simulink library "LibraryFM"  (R2016b)
settings: Solver=VariableStepAuto  StartTime=0.0  StopTime=10.0  RelTol=1e-3
undefined symbols (not defined in the file or in its folder): ActuatorStruct, drivePeakCurrent, FM1, Lb, Lf, Lu, motorTorqueConstant, RobotStruct, sampleTime, transmissionRatio
undefined symbols (not defined in the file): JointAbsoluteEncoderCounts_rev
libraries: simulink x34, LibraryFM x13, VariousBlocksLibrary x4, dspstat3 x1, simulink_extras x1, FM_Library x1
(part 2 of 3)

== system LibraryFM/DataToEtherCAT/WorkspacePositionGuard ==
  note: Check for singularity of joint configuration by checking
      | the condition number. When it exceeds a certain value, go to a safe mode
      | For now, this means disabling the actuators.
      | Note that the boundaries set using admittance should prohibit this from happening.
      | However, if sometjhing really goes wrong, this is a safe guard
  note: Check whether endpoint position is within the predefined workspace
      | (ellipse)
  note: Check internal angles
  BusRobot : Inport
  StateSystem : Inport  Port=2
  AvoidAlgebraicLoop : Memory
  Bus Selector : BusSelector  OutputSignals=xOpSpace.x,xOpSpace.jacobian,qJointSpace.q_all
  CheckForSingularity : MATLAB Function  TreatAsAtomicUnit=on
  CheckInternalAngles : MATLAB Function  TreatAsAtomicUnit=on
  Compare To Constant : simulink/Logic and Bit Operations/Compare To Constant  relop===  const=4  OutDataTypeStr=boolean
  Compare To Constant1 : simulink/Logic and Bit Operations/Compare To Constant  relop=>=  const=120  OutDataTypeStr=boolean
  CreateSingleErrorValue : LibraryFM/ToActuator1/DriveEnableLogic/CreateSingleErrorValue
  Data Type Conversion1 : DataTypeConversion  OutDataTypeStr=boolean
  Data Type Conversion2 : DataTypeConversion  Commented=through  OutDataTypeStr=int32
  Data Type Conversion4 : DataTypeConversion  OutDataTypeStr=boolean
  Detect Change : simulink/Logic and Bit Operations/Detect Change  vinit=0  InputProcessing=Inherited  OutDataTypeStr=boolean
  EndpointPositionGuard : MATLAB Function  TreatAsAtomicUnit=on
  LatchRising : LibraryFM/Utilities/LatchRising  ic=0
  Mux : Mux  Inputs=3
  ShowWorkspaceErrorLatched : Display
  WorkspaceLastError : Display
  WorkspaceError : Outport
  WorkspaceErrorLatched : Outport  Port=2
  wires:
  Data Type Conversion4/1 -> Mux/3
  Bus Selector/3 -> CheckInternalAngles/1(theta)  "<q_all>"
  CheckInternalAngles/1(angleError) -> Data Type Conversion4/1
  Compare To Constant1/1 -> Mux/2
  Data Type Conversion1/1 -> Mux/1
  Data Type Conversion2/1 -> WorkspaceErrorLatched/1, ShowWorkspaceErrorLatched/1
  StateSystem/1 -> Compare To Constant/1
  Bus Selector/2 -> CheckForSingularity/1(J)  "<jacobian>"
  Compare To Constant/1 -> EndpointPositionGuard/2(correctState)
  AvoidAlgebraicLoop/1 -> WorkspaceError/1, Detect Change/1, LatchRising/1
  Detect Change/1 -> LatchRising/Trigger
  CreateSingleErrorValue/1 -> AvoidAlgebraicLoop/1
  EndpointPositionGuard/1(error) -> Data Type Conversion1/1
  LatchRising/1 -> Data Type Conversion2/1
  Bus Selector/1 -> EndpointPositionGuard/1(xe)  "<x>"
  BusRobot/1 -> Bus Selector/1
  Mux/1 -> WorkspaceLastError/1, CreateSingleErrorValue/1
  CheckForSingularity/1(kappa) -> Compare To Constant1/1

== system LibraryFM/DriveEnableLogic1/16_TorqueGuard ==
  BusActuator : Inport
  TorqueGuardMax : Inport  Port=2
  Abs : Abs
  Bus Selector : BusSelector  OutputSignals=JointTorque_Act_Nm
  Relational Operator : RelationalOperator  Operator=>  OutDataTypeStr=boolean  RndMeth=Nearest
  Error : Outport
  wires:
  Relational Operator/1 -> Error/1
  Abs/1 -> Relational Operator/1
  BusActuator/1 -> Bus Selector/1
  Bus Selector/1 -> Abs/1  "<JointTorque_Act_Nm>"
  TorqueGuardMax/1 -> Relational Operator/2

== system LibraryFM/DriveEnableLogic1/1_ActuatorNotInUse ==
  note: When UseActuator = 0, this block outputs 1. Later in the chain, the ErrorValue is then negated, resulting in -1 if there are no other errors. Note, thus, that this output does not really indicate an error; more a status.
  UseActuator : Inport
  Logical Operator1 : Logic  Operator=NOT  AllPortsSameDT=off  OutDataTypeStr=boolean
  Error : Outport
  wires:
  UseActuator/1 -> Logical Operator1/1
  Logical Operator1/1 -> Error/1

== system LibraryFM/DriveEnableLogic1/2_JointAnglePositionGuard ==
  note: This block makes sure that the motors are turned off (and cannot go on) when the joint is outside its normal range.
  BusActuator : Inport
  Bus Selector : BusSelector  OutputSignals=JointPosition_rad
  Logical Operator : Logic  Operator=OR  AllPortsSameDT=off  OutDataTypeStr=boolean
  Maximum : Constant  Value=ActuatorStruct.JointPositionGuardMax
  Minimum : Constant  Value=ActuatorStruct.JointPositionGuardMin
  Relational Operator : RelationalOperator  Operator=<=  OutDataTypeStr=boolean  RndMeth=Nearest
  Relational Operator1 : RelationalOperator  OutDataTypeStr=boolean  RndMeth=Nearest
  Error : Outport
  wires:
  Bus Selector/1 -> Relational Operator/1, Relational Operator1/1  "<JointPosition_rad>"
  Maximum/1 -> Relational Operator1/2
  Minimum/1 -> Relational Operator/2
  Logical Operator/1 -> Error/1
  Relational Operator1/1 -> Logical Operator/2
  Relational Operator/1 -> Logical Operator/1
  BusActuator/1 -> Bus Selector/1

== system LibraryFM/DriveEnableLogic1/32_DriveError ==
  note: This block checks whether the drive went off by itself. Reasons why this could happen are: undervoltage of the motor power supply, short-circuit detection triggered, I2t error etc.
      | The first few seconds that the drive should be on (i.e., DriveEnable = True), the drive is in the process of turning on, and will not be really on. In order to avoid direct turn-off due to this, we disable this error the first few seconds.
  note: This memory block is to avoid an
      | algebraic loop
  note: This memory block is to avoid that this error 'turns on' when another error is triggered.
  BusActuator : Inport
  DriveEnable : Inport  Port=2
  Bus Selector : BusSelector  OutputSignals=OperationEnabled
  CountHowLongEnableWasTrue : MATLAB Function  TreatAsAtomicUnit=on
  InhibitTime_s : Constant  Value=2.0
  Logical Operator : Logic  AllPortsSameDT=off  OutDataTypeStr=boolean
  Logical Operator2 : Logic  Operator=NOT  AllPortsSameDT=off  OutDataTypeStr=boolean
  Memory : Memory
  Memory1 : Memory
  Relational Operator : RelationalOperator  OutDataTypeStr=boolean  RndMeth=Nearest
  ToSeconds : Gain  Gain=sampleTime
  Error : Outport
  wires:
  Logical Operator2/1 -> Logical Operator/2
  Memory1/1 -> Bus Selector/1
  Memory/1 -> CountHowLongEnableWasTrue/1(u)
  InhibitTime_s/1 -> Relational Operator/2
  Relational Operator/1 -> Logical Operator/1
  ToSeconds/1 -> Relational Operator/1
  CountHowLongEnableWasTrue/1(y) -> ToSeconds/1
  DriveEnable/1 -> Memory/1
  Bus Selector/1 -> Logical Operator2/1  "<OperationEnabled>"
  BusActuator/1 -> Memory1/1
  Logical Operator/1 -> Error/1

== system LibraryFM/DriveEnableLogic1/4_TransmissionSlip ==
  note: This block makes sure that the motors are turned off when the transmission slips.
  BusActuator : Inport
  Abs : Abs
  Bus Selector : BusSelector  OutputSignals=JointPosition_rad,JointPosition_AbsEnc_rad
  Minimum : Constant  Value=ActuatorStruct.TransmissionSlipAngleGuardMax
  Relational Operator1 : RelationalOperator  OutDataTypeStr=boolean  RndMeth=Nearest
  Slip : Display
  Subtract : Sum  Inputs=+-
  Error : Outport
  wires:
  Abs/1 -> Relational Operator1/1
  Bus Selector/1 -> Subtract/1  "<JointPosition_rad>"
  BusActuator/1 -> Bus Selector/1
  Minimum/1 -> Relational Operator1/2
  Bus Selector/2 -> Subtract/2  "<JointPosition_AbsEnc_rad>"
  Subtract/1 -> Abs/1, Slip/1
  Relational Operator1/1 -> Error/1

== system LibraryFM/DriveEnableLogic1/8_JointVelocityGuard ==
  To_ToActuator : Inport
  Abs : Abs
  Bus Selector : BusSelector  OutputSignals=JointPosition_rad
  Constant : Constant  Value=2*pi
  LPF Diff : Subsystem
  Relational Operator : RelationalOperator  OutDataTypeStr=boolean  RndMeth=Simplest
  Error : Outport
  wires:
  To_ToActuator/1 -> Bus Selector/1
  Bus Selector/1 -> LPF Diff/1(JointPosition_rad)  "<JointPosition_rad>"
  LPF Diff/1(JointVelocity_LPF_rads) -> Abs/1
  Abs/1 -> Relational Operator/1
  Constant/1 -> Relational Operator/2
  Relational Operator/1 -> Error/1

== system LibraryFM/DriveEnableLogic1/LatchRising ==
  in : Inport
  Trigger : TriggerPort  VariantControl=Variant  PortDimensions=1
  out : Outport
  wires:
  in/1 -> out/1

== system LibraryFM/FromActuator1/CalculateJointVelocity ==
  JointPosition_rad : Inport
  FOAW : MATLAB Function  Commented=on  TreatAsAtomicUnit=on
  Gain : Gain  Commented=on
  LPF Diff - 2nd order : LibraryFM/LPF Diff - 2nd order
  encoder noise : Constant  Commented=on  Value=ActuatorStruct.FOAWNoiseLevel
  JointVelocity_rads : Outport
  JointVelocity_LPF_rads : Outport  Port=2
  wires:
  JointPosition_rad/1 -> LPF Diff - 2nd order/1
  LPF Diff - 2nd order/1 -> JointVelocity_rads/1, JointVelocity_LPF_rads/1
  encoder noise/1 -> Gain/1
  Gain/1 -> FOAW/2(noise)

== system LibraryFM/PD + AFFC/AFFC ==
  q_ref : Inport
  qdot_ref : Inport  Port=2
  qddot_ref : Inport  Port=3
  e : Inport  Port=4
  Enable : EnablePort  StatesWhenEnabling=reset
  AFFC : MATLAB Function  TreatAsAtomicUnit=on
  Counter Free-Running : simulink/Sources/Counter Free-Running  NumBits=32  tsamp=-1
  Data Type Conversion : DataTypeConversion  OutDataTypeStr=double
  Learning factors : Constant  Value=[1e-5;5e-3;5e-4;1e-3]
  sample time : Gain  Gain=sampleTime
  p : Outport  OutputWhenDisabled=reset  InitialOutput=zeros(7,1)
  tau_affc : Outport  Port=2  OutputWhenDisabled=reset  InitialOutput=[0;0]
  wires:
  Learning factors/1 -> AFFC/6(w)
  Data Type Conversion/1 -> sample time/1
  sample time/1 -> AFFC/1(t)
  Counter Free-Running/1 -> Data Type Conversion/1
  AFFC/1(p) -> p/1
  AFFC/2(tau) -> tau_affc/1
  q_ref/1 -> AFFC/2(q)
  qdot_ref/1 -> AFFC/3(qdot)
  qddot_ref/1 -> AFFC/4(qddot)
  e/1 -> AFFC/5(e)

== system LibraryFM/ToActuator1/AppendToBus ==
  Bus_in : Inport
  DriveError : Inport  Port=2
  DesiredTorque : Inport  Port=3
  DesiredTorqueLimited : Inport  Port=4
  Bus Creator : BusCreator  Inputs=12
  Bus Selector2 : BusSelector  OutputSignals=OperationEnabled,StatusWord,JointPosition_IncEnc_rad,JointVelocity_LPF_rads,MotorEncoder_counts,MotorPosition_IncEnc_rad,JointAbsoluteEncoder_counts,JointTorque_Act_Nm,JointPosition_AbsEnc_rad
  Data Type Conversion : DataTypeConversion  OutDataTypeStr=double
  Bus_out : Outport
  wires:
  Bus Selector2/8 -> Bus Creator/8  "<JointTorque_Act_Nm>"
  Bus Creator/1 -> Bus_out/1
  Bus_in/1 -> Bus Selector2/1
  DriveError/1 -> Data Type Conversion/1
  Data Type Conversion/1 -> Bus Creator/12  "DriveError"
  DesiredTorque/1 -> Bus Creator/10  "DesiredTorque_Nm"
  DesiredTorqueLimited/1 -> Bus Creator/11  "DesiredTorqueLimited_Nm"
  Bus Selector2/1 -> Bus Creator/1  "<OperationEnabled>"
  Bus Selector2/2 -> Bus Creator/2  "<StatusWord>"
  Bus Selector2/3 -> Bus Creator/3  "<JointPosition_IncEnc_rad>"
  Bus Selector2/4 -> Bus Creator/4  "<JointVelocity_LPF_rads>"
  Bus Selector2/5 -> Bus Creator/5  "<MotorEncoder_counts>"
  Bus Selector2/7 -> Bus Creator/7  "<JointAbsoluteEncoder_counts>"
  Bus Selector2/6 -> Bus Creator/6  "<MotorPosition_IncEnc_rad>"
  Bus Selector2/9 -> Bus Creator/9  "<JointPosition_AbsEnc_rad>"

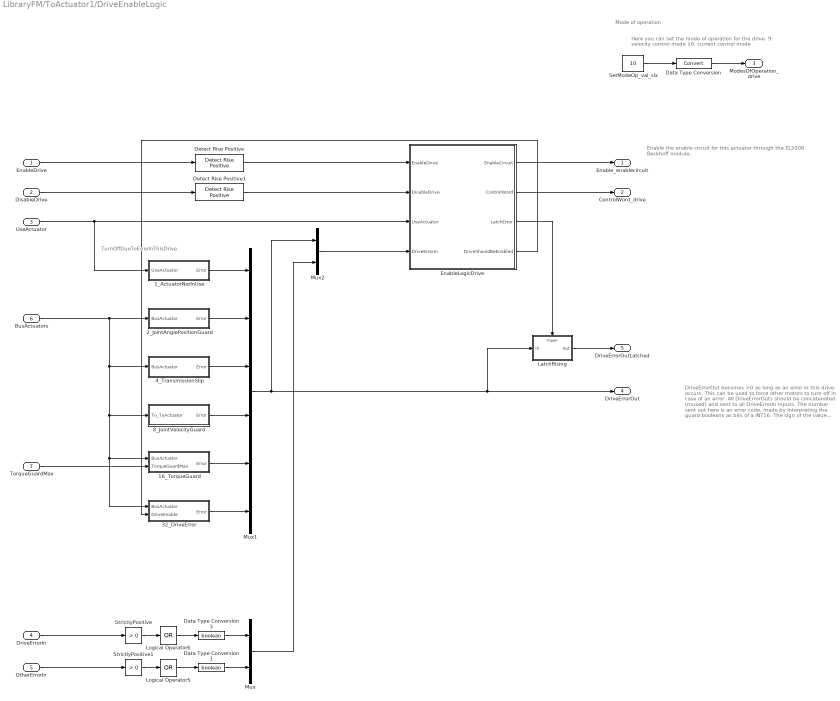
== system LibraryFM/ToActuator1/DriveEnableLogic ==
  note: Mode of operation
  note: Here you can set the mode of operation for the drive.
      | 9: velocity control mode
      | 10: current control mode
  note: TurnOffDueToErrorInThisDrive
  note: DriveErrorOut becomes >0 as long as an error in this drive occurs. This can be used to force other motors to turn off in case of an error.
      | All DriveErrorOuts should be concatenated (muxed)  and sent to all DriveErrorIn inputs. The number sent out here is an error code, made by interpreting the guard booleans as bits of a INT16.
      | The sign of the value indicates:
      | >=0: UseActuator=true
      | <0: UseActuator = False
  note: Enable the enable circuit for this actuator through the EL2008
      | Beckhoff module.
  EnableDrive : Inport
  DisableDrive : Inport  Port=2
  UseActuator : Inport  Port=3
  DriveErrorIn : Inport  Port=4
  OtherErrorIn : Inport  Port=5
  BusActuators : Inport  Port=6
  TorqueGuardMax : Inport  Port=7
  16_TorqueGuard : Subsystem
  1_ActuatorNotInUse : Subsystem
  2_JointAnglePositionGuard : Subsystem
  32_DriveError : Subsystem
  4_TransmissionSlip : Subsystem
  8_JointVelocityGuard : Subsystem
  Data Type Conversion : DataTypeConversion
  Data Type Conversion1 : DataTypeConversion  OutDataTypeStr=boolean
  Data Type Conversion3 : DataTypeConversion  OutDataTypeStr=boolean
  Detect Rise Positive : simulink/Logic and Bit Operations/Detect Rise Positive  vinit=0  InputProcessing=Inherited  OutDataTypeStr=boolean
  Detect Rise Positive1 : simulink/Logic and Bit Operations/Detect Rise Positive  vinit=0  InputProcessing=Inherited  OutDataTypeStr=boolean
  EnableLogicDrive : Subsystem
  LatchRising : Subsystem  TreatAsAtomicUnit=on
  Logical Operator5 : Logic  Operator=OR  Inputs=1  AllPortsSameDT=off  OutDataTypeStr=boolean
  Logical Operator6 : Logic  Operator=OR  Inputs=1  AllPortsSameDT=off  OutDataTypeStr=boolean
  Mux : Mux  Inputs=2
  Mux1 : Mux  Inputs=6
  Mux2 : Mux  Inputs=2
  SetModeOp_val_slx : Constant  Value=10
  StrictlyPositive : simulink/Logic and Bit Operations/Compare To Zero  relop=>  OutDataTypeStr=boolean
  StrictlyPositive1 : simulink/Logic and Bit Operations/Compare To Zero  relop=>  OutDataTypeStr=boolean
  Enable_enablecircuit : Outport
  ControlWord_drive : Outport  Port=2
  ModesOfOperation_drive : Outport  Port=3
  DriveErrorOut : Outport  Port=4
  DriveErrorOutLatched : Outport  Port=5
  wires:
  Mux/1 -> Mux2/2
  OtherErrorIn/1 -> StrictlyPositive1/1
  Logical Operator5/1 -> Data Type Conversion1/1
  Data Type Conversion3/1 -> Mux/1
  16_TorqueGuard/1(Error) -> Mux1/5
  32_DriveError/1(Error) -> Mux1/6
  1_ActuatorNotInUse/1(Error) -> Mux1/1
  BusActuators/1 -> 4_TransmissionSlip/1(BusActuator), 8_JointVelocityGuard/1(To_ToActuator), 32_DriveError/1(BusActuator), 16_TorqueGuard/1(BusActuator), 2_JointAnglePositionGuard/1(BusActuator)
  Logical Operator6/1 -> Data Type Conversion3/1
  DriveErrorIn/1 -> StrictlyPositive/1
  UseActuator/1 -> 1_ActuatorNotInUse/1(UseActuator), EnableLogicDrive/3(UseActuator)
  Data Type Conversion/1 -> ModesOfOperation_drive/1
  DisableDrive/1 -> Detect Rise Positive1/1
  Detect Rise Positive1/1 -> EnableLogicDrive/2(DisableDrive)
  EnableDrive/1 -> Detect Rise Positive/1
  SetModeOp_val_slx/1 -> Data Type Conversion/1
  TorqueGuardMax/1 -> 16_TorqueGuard/2(TorqueGuardMax)
  StrictlyPositive/1 -> Logical Operator6/1
  Mux1/1 -> DriveErrorOut/1, LatchRising/1(in), Mux2/1
  4_TransmissionSlip/1(Error) -> Mux1/3
  2_JointAnglePositionGuard/1(Error) -> Mux1/2
  LatchRising/1(out) -> DriveErrorOutLatched/1
  8_JointVelocityGuard/1(Error) -> Mux1/4
  Detect Rise Positive/1 -> EnableLogicDrive/1(EnableDrive)
  Mux2/1 -> EnableLogicDrive/4(DriveErrorIn)
  EnableLogicDrive/1(EnableCircuit) -> Enable_enablecircuit/1
  EnableLogicDrive/2(ControlWord) -> ControlWord_drive/1
  EnableLogicDrive/3(LatchError) -> LatchRising/Trigger
  EnableLogicDrive/4(DriveShouldBeEnabled) -> 32_DriveError/2(DriveEnable)
  StrictlyPositive1/1 -> Logical Operator5/1
  Data Type Conversion1/1 -> Mux/2

== system LibraryFM/Utilities/CrossFade ==
  In1 : Inport
  In2 : Inport  Port=2
  AmountIn2 : Inport  Port=3
  Add : Sum  Inputs=+-
  Add1 : Sum
  One : Constant
  Product : Product  RndMeth=Zero
  Product1 : Product  RndMeth=Zero
  Saturation : Saturate  UpperLimit=1  LowerLimit=0
  Out : Outport
  wires:
  In1/1 -> Product1/1
  AmountIn2/1 -> Saturation/1
  One/1 -> Add/1
  Saturation/1 -> Product/2, Add/2
  Add/1 -> Product1/2
  Product/1 -> Add1/2
  Product1/1 -> Add1/1
  In2/1 -> Product/1
  Add1/1 -> Out/1

== system LibraryFM/Utilities/Cycloid ==
  note: Given a linear input 0<=in<=1, it gives a cycloid output 0<=out<=1.
      | If In is outside the 0..1 range, it is limited to 0 or 1.
  In : Inport
  Gain1 : Gain  Gain=2*pi
  Gain2 : Gain  Gain=1/(2*pi)
  Saturation : Saturate  UpperLimit=1  LowerLimit=0
  Subtract : Sum  Inputs=+-
  Trigonometric Function : Trigonometry
  Out : Outport
  wires:
  Gain1/1 -> Trigonometric Function/1
  Subtract/1 -> Out/1
  In/1 -> Saturation/1
  Saturation/1 -> Gain1/1, Subtract/1
  Trigonometric Function/1 -> Gain2/1
  Gain2/1 -> Subtract/2

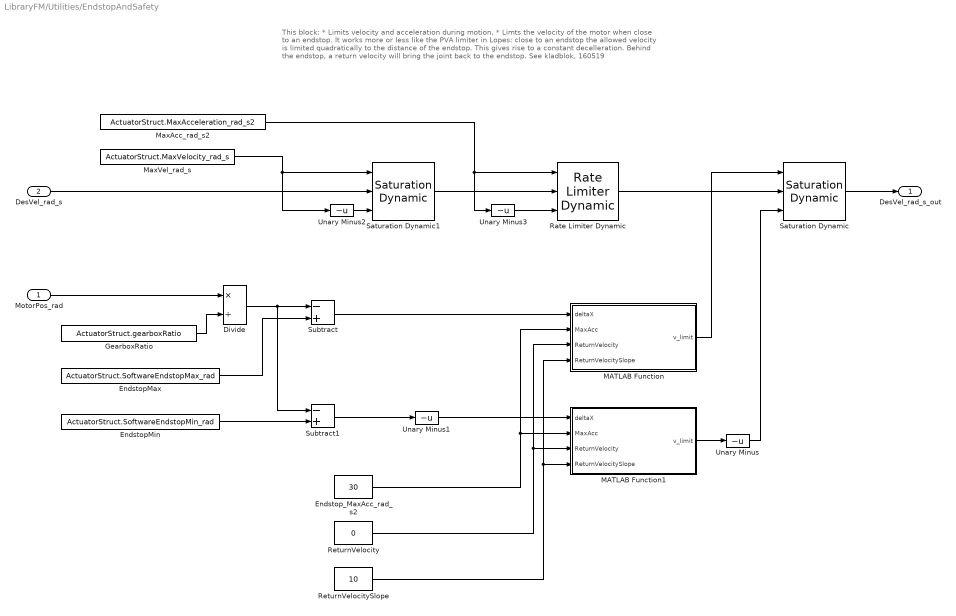
== system LibraryFM/Utilities/EndstopAndSafety ==
  note: This block:
      | * Limits velocity and acceleration during motion,
      | * Limts the velocity of the motor when close to an endstop. It works more or less like the PVA limiter in Lopes: close to an endstop the allowed velocity is limited quadratically to the distance of the endstop. This gives rise to a constant decelleration. Behind the endstop, a return velocity will bring the joint back to the endstop.  See kladblok, 160519
  MotorPos_rad : Inport
  DesVel_rad_s : Inport  Port=2
  Divide : Product  Inputs=*/
  EndstopMax : Constant  Value=ActuatorStruct.SoftwareEndstopMax_rad
  EndstopMin : Constant  Value=ActuatorStruct.SoftwareEndstopMin_rad
  Endstop_MaxAcc_rad_s2 : Constant  Value=30
  GearboxRatio : Constant  Value=ActuatorStruct.gearboxRatio
  MATLAB Function : MATLAB Function  TreatAsAtomicUnit=on
  MATLAB Function1 : MATLAB Function  TreatAsAtomicUnit=on
  MaxAcc_rad_s2 : Constant  Value=ActuatorStruct.MaxAcceleration_rad_s2
  MaxVel_rad_s : Constant  Value=ActuatorStruct.MaxVelocity_rad_s
  Rate Limiter Dynamic : simulink/Discontinuities/Rate Limiter Dynamic
  ReturnVelocity : Constant  Value=0
  ReturnVelocitySlope : Constant  Value=10
  Saturation Dynamic : simulink/Discontinuities/Saturation Dynamic  OutMin=[]  OutMax=[]  OutDataTypeStr=Inherit: Same as second input  OutDataType=fixdt(1, 16)  OutScaling=2^-10  DoSatur=off
  Saturation Dynamic1 : simulink/Discontinuities/Saturation Dynamic  OutMin=[]  OutMax=[]  OutDataTypeStr=Inherit: Same as second input  OutDataType=fixdt(1, 16)  OutScaling=2^-10  DoSatur=off
  Subtract : Sum  Inputs=-+
  Subtract1 : Sum  Inputs=-+
  Unary Minus{,1..3} (4 alike) : UnaryMinus
  DesVel_rad_s_out : Outport
  wires:
  Unary Minus3/1 -> Rate Limiter Dynamic/3
  MaxAcc_rad_s2/1 -> Rate Limiter Dynamic/1, Unary Minus3/1
  Unary Minus2/1 -> Saturation Dynamic1/3
  MaxVel_rad_s/1 -> Saturation Dynamic1/1, Unary Minus2/1
  DesVel_rad_s/1 -> Saturation Dynamic1/2
  Saturation Dynamic1/1 -> Rate Limiter Dynamic/2
  Rate Limiter Dynamic/1 -> Saturation Dynamic/2
  MotorPos_rad/1 -> Divide/1
  GearboxRatio/1 -> Divide/2
  Divide/1 -> Subtract1/1, Subtract/1
  EndstopMax/1 -> Subtract/2
  ReturnVelocitySlope/1 -> MATLAB Function1/4(ReturnVelocitySlope), MATLAB Function/4(ReturnVelocitySlope)
  ReturnVelocity/1 -> MATLAB Function1/3(ReturnVelocity), MATLAB Function/3(ReturnVelocity)
  MATLAB Function/1(v_limit) -> Saturation Dynamic/1
  MATLAB Function1/1(v_limit) -> Unary Minus/1
  Subtract1/1 -> Unary Minus1/1
  EndstopMin/1 -> Subtract1/2
  Endstop_MaxAcc_rad_s2/1 -> MATLAB Function1/2(MaxAcc), MATLAB Function/2(MaxAcc)
  Subtract/1 -> MATLAB Function/1(deltaX)
  Unary Minus/1 -> Saturation Dynamic/3
  Unary Minus1/1 -> MATLAB Function1/1(deltaX)
  Saturation Dynamic/1 -> DesVel_rad_s_out/1

== system LibraryFM/Utilities/FilterFourthOrder ==
  In : Inport
  Omega : Inport  Port=2
  Filter1 : MATLAB Function  TreatAsAtomicUnit=on  mask{sampleTime=sampleTime}
      mask prompts: sampleTime "Sample Time"
  Filter2 : MATLAB Function  TreatAsAtomicUnit=on  mask{sampleTime=sampleTime}
      mask prompts: sampleTime "Sample Time"
  Out : Outport
  wires:
  Filter2/1(y) -> Out/1
  In/1 -> Filter1/1(x)
  Omega/1 -> Filter1/2(OmegaFilter), Filter2/2(OmegaFilter)
  Filter1/1(y) -> Filter2/1(x)

== system LibraryFM/Utilities/Latch ==
  note: Enable == HIGH: OUtput follows input
      | Enable == LOW: Output does not change anymore.
  In : Inport
  Enable : EnablePort
  Out : Outport  InitialOutput=ic
  wires:
  In/1 -> Out/1

== system LibraryFM/Utilities/LatchRising ==
  note: Enable == HIGH: OUtput follows input
      | Enable == LOW: Output does not change anymore.
  In : Inport
  Trigger : TriggerPort  VariantControl=Variant  PortDimensions=1
  Out : Outport  InitialOutput=ic
  wires:
  In/1 -> Out/1

== system LibraryFM/Utilities/Stopwatch ==
  note: Stopwatch -
      | Outputs time in seconds.
      | Reset during high level of Rest pulse
  ResetHighActive : Inport
  Counter Free-Running : simulink/Sources/Counter Free-Running  NumBits=32  tsamp=-1
  Data Type Conversion : DataTypeConversion  OutDataTypeStr=double
  LatchRising : FM_Library/LatchRising  ic=0
  Subtract : Sum  Inputs=-+
  sample time : Gain  Gain=sampleTime
  Time_s : Outport
  wires:
  ResetHighActive/1 -> LatchRising/Trigger
  Data Type Conversion/1 -> sample time/1
  sample time/1 -> Time_s/1
  Subtract/1 -> Data Type Conversion/1
  Counter Free-Running/1 -> LatchRising/1, Subtract/2
  LatchRising/1 -> Subtract/1  "startTime"

== system LibraryFM/Utilities/TorqueLimiter ==
  note: This block limits the Desird Torque to an interval [-TorqueLimit, +TorqueLimit]. It also sets TorqueGuardMax_Nm to 0.5 Nm more than the TorqueLimit. This is used in the DriveEnableLogic block to completely shut down the motor (and with that, all other motors) if the limit is severly (by 0.5 Nm) exceeded.
      |
      | Note that the actuators are rated to a maximum of 4 Nm, so if the user puts a TorqueLimit of higher than 4 Nm in, this block will still limit it to 4 Nm.
  Torque_Limit_Nm : Inport
  Torque_Des_Nm : Inport  Port=2
  AbsoluteMaximumTorque_Nm : Constant  Value=8
  Bias : Bias  Bias=0.5
  MinMax : MinMax  Inputs=2
  Saturation Dynamic : simulink/Discontinuities/Saturation Dynamic  OutMin=[]  OutMax=[]  OutDataTypeStr=Inherit: Same as second input  OutDataType=fixdt(1, 16)  OutScaling=2^-10  DoSatur=off
  Unary Minus : UnaryMinus
  Torque_GuardMax_Nm : Outport
  Torque_Des_Limited_Nm : Outport  Port=2
  wires:
  Torque_Limit_Nm/1 -> MinMax/1
  AbsoluteMaximumTorque_Nm/1 -> MinMax/2
  MinMax/1 -> Bias/1, Unary Minus/1, Saturation Dynamic/1
  Unary Minus/1 -> Saturation Dynamic/3
  Saturation Dynamic/1 -> Torque_Des_Limited_Nm/1
  Torque_Des_Nm/1 -> Saturation Dynamic/2
  Bias/1 -> Torque_GuardMax_Nm/1

== system LibraryFM/DataFromEtherCAT/Calculate Arrange Joint and Op Space/forward kinematics ==
  JointPosition_rad : Inport  PortDimensions=[2 1]
  JointVelocity_rads : Inport  Port=2  PortDimensions=[2 1]
  JointAcceleration_rads2 : Inport  Port=3  PortDimensions=[2 1]
  Je : MATLAB Function  TreatAsAtomicUnit=on
  Jedot : MATLAB Function  TreatAsAtomicUnit=on
  Product : Product  Multiplication=Matrix(*)
  calculate xddot : MATLAB Function  TreatAsAtomicUnit=on
  forward kinematics : MATLAB Function  TreatAsAtomicUnit=on
  x : Outport
  xdot : Outport  Port=2
  xddot : Outport  Port=3
  J : Outport  Port=4
  Jdot : Outport  Port=5
  wires:
  JointAcceleration_rads2/1 -> calculate xddot/1(qddot)
  calculate xddot/1(xddot) -> xddot/1
  forward kinematics/1(x) -> x/1
  Product/1 -> xdot/1
  Jedot/1(Jedot) -> Jdot/1, calculate xddot/4(Jdot)
  JointVelocity_rads/1 -> Jedot/2(qdot), Product/2, calculate xddot/2(qdot)
  Je/1(Je) -> J/1, Product/1, calculate xddot/3(J)
  JointPosition_rad/1 -> Je/1(q), Jedot/1(q), forward kinematics/1(q)

== system LibraryFM/DriveEnableLogic1/8_JointVelocityGuard/LPF Diff ==
  JointPosition_rad : Inport
  Discrete Derivative : simulink/Discrete/Discrete Derivative  gainval=1.0  ICPrevScaledInput=0.0  InputProcessing=Inherited  OutMin=[]  OutMax=[]  OutDataType=fixdt(1, 16)  OutScaling=2^-10  DoSatur=off
  Freq [Hz] : Constant  Value=100  OutDataTypeStr=double
  MATLAB Function : MATLAB Function  TreatAsAtomicUnit=on
  Unit Delay : UnitDelay  SampleTime=-1
  JointVelocity_LPF_rads : Outport
  wires:
  Discrete Derivative/1 -> MATLAB Function/1(u)
  MATLAB Function/1(y) -> JointVelocity_LPF_rads/1, Unit Delay/1
  JointPosition_rad/1 -> Discrete Derivative/1
  Unit Delay/1 -> MATLAB Function/3(y_prev)
  Freq [Hz]/1 -> MATLAB Function/2(freq)

== system LibraryFM/ToActuator1/DriveEnableLogic/16_TorqueGuard ==
  BusActuator : Inport
  TorqueGuardMax : Inport  Port=2
  Abs : Abs
  Bus Selector : BusSelector  OutputSignals=JointTorque_Act_Nm
  Relational Operator : RelationalOperator  Operator=>  OutDataTypeStr=boolean  RndMeth=Nearest
  Error : Outport
  wires:
  Relational Operator/1 -> Error/1
  Abs/1 -> Relational Operator/1
  BusActuator/1 -> Bus Selector/1
  Bus Selector/1 -> Abs/1  "<JointTorque_Act_Nm>"
  TorqueGuardMax/1 -> Relational Operator/2

== system LibraryFM/ToActuator1/DriveEnableLogic/1_ActuatorNotInUse ==
  note: When UseActuator = 0, this block outputs 1. Later in the chain, the ErrorValue is then negated, resulting in -1 if there are no other errors. Note, thus, that this output does not really indicate an error; more a status.
  UseActuator : Inport
  Logical Operator1 : Logic  Operator=NOT  AllPortsSameDT=off  OutDataTypeStr=boolean
  Error : Outport
  wires:
  UseActuator/1 -> Logical Operator1/1
  Logical Operator1/1 -> Error/1

== system LibraryFM/ToActuator1/DriveEnableLogic/2_JointAnglePositionGuard ==
  note: This block makes sure that the motors are turned off (and cannot go on) when the joint is outside its normal range.
  BusActuator : Inport
  Bus Selector : BusSelector  OutputSignals=JointPosition_IncEnc_rad
  Logical Operator : Logic  Operator=OR  AllPortsSameDT=off  OutDataTypeStr=boolean
  Maximum : Constant  Value=ActuatorStruct.JointPositionGuardMax
  Minimum : Constant  Value=ActuatorStruct.JointPositionGuardMin
  Relational Operator : RelationalOperator  Operator=<=  OutDataTypeStr=boolean  RndMeth=Nearest
  Relational Operator1 : RelationalOperator  OutDataTypeStr=boolean  RndMeth=Nearest
  Error : Outport
  wires:
  Bus Selector/1 -> Relational Operator/1, Relational Operator1/1  "<JointPosition_IncEnc_rad>"
  Maximum/1 -> Relational Operator1/2
  Minimum/1 -> Relational Operator/2
  Logical Operator/1 -> Error/1
  Relational Operator1/1 -> Logical Operator/2
  Relational Operator/1 -> Logical Operator/1
  BusActuator/1 -> Bus Selector/1

== system LibraryFM/ToActuator1/DriveEnableLogic/32_DriveError ==
  note: This block checks whether the drive went off by itself. Reasons why this could happen are: undervoltage of the motor power supply, short-circuit detection triggered, I2t error etc.
      | The first few seconds that the drive should be on (i.e., DriveEnable = True), the drive is in the process of turning on, and will not be really on. In order to avoid direct turn-off due to this, we disable this error the first few seconds.
  note: This memory block is to avoid an
      | algebraic loop
  note: This memory block is to avoid that this error 'turns on' when another error is triggered.
  BusActuator : Inport
  DriveEnable : Inport  Port=2
  Bus Selector : BusSelector  OutputSignals=OperationEnabled
  CountHowLongEnableWasTrue : MATLAB Function  TreatAsAtomicUnit=on
  InhibitTime_s : Constant  Value=2.0
  Logical Operator : Logic  AllPortsSameDT=off  OutDataTypeStr=boolean
  Logical Operator2 : Logic  Operator=NOT  AllPortsSameDT=off  OutDataTypeStr=boolean
  Memory : Memory
  Memory1 : Memory
  Relational Operator : RelationalOperator  OutDataTypeStr=boolean  RndMeth=Nearest
  ToSeconds : Gain  Gain=sampleTime
  Error : Outport
  wires:
  Logical Operator2/1 -> Logical Operator/2
  Memory1/1 -> Bus Selector/1
  Memory/1 -> CountHowLongEnableWasTrue/1(u)
  InhibitTime_s/1 -> Relational Operator/2
  Relational Operator/1 -> Logical Operator/1
  ToSeconds/1 -> Relational Operator/1
  CountHowLongEnableWasTrue/1(y) -> ToSeconds/1
  DriveEnable/1 -> Memory/1
  Bus Selector/1 -> Logical Operator2/1  "<OperationEnabled>"
  BusActuator/1 -> Memory1/1
  Logical Operator/1 -> Error/1

== system LibraryFM/ToActuator1/DriveEnableLogic/4_TransmissionSlip ==
  note: This block makes sure that the motors are turned off when the transmission slips.
  BusActuator : Inport
  Abs : Abs
  Bus Selector : BusSelector  OutputSignals=JointPosition_IncEnc_rad,JointPosition_AbsEnc_rad
  MinMax Running Resettable : simulink/Math Operations/MinMax Running Resettable  Function=min  vinit=0.0
  Minimum : Constant  Value=ActuatorStruct.TransmissionSlipAngleGuardMax
  Minimum1 : Constant  Value=0
  Relational Operator1 : RelationalOperator  OutDataTypeStr=boolean  RndMeth=Nearest
  Slip : Display
  Slip1 : Display
  Subtract : Sum  Inputs=+-
  Error : Outport
  wires:
  Abs/1 -> Relational Operator1/1
  Bus Selector/1 -> Subtract/1  "<JointPosition_IncEnc_rad>"
  BusActuator/1 -> Bus Selector/1
  Minimum/1 -> Relational Operator1/2
  Bus Selector/2 -> Subtract/2  "<JointPosition_AbsEnc_rad>"
  Subtract/1 -> Abs/1, MinMax Running Resettable/1, Slip/1
  Relational Operator1/1 -> Error/1
  MinMax Running Resettable/1 -> Slip1/1
  Minimum1/1 -> MinMax Running Resettable/2

== system LibraryFM/ToActuator1/DriveEnableLogic/8_JointVelocityGuard ==
  To_ToActuator : Inport
  Abs : Abs
  Bus Selector : BusSelector  OutputSignals=JointPosition_IncEnc_rad
  Constant : Constant  Value=6*pi
  LPF Diff : Subsystem
  Relational Operator : RelationalOperator  OutDataTypeStr=boolean  RndMeth=Simplest
  Error : Outport
  wires:
  To_ToActuator/1 -> Bus Selector/1
  Bus Selector/1 -> LPF Diff/1(JointPosition_rad)  "<JointPosition_IncEnc_rad>"
  LPF Diff/1(JointVelocity_LPF_rads) -> Abs/1
  Abs/1 -> Relational Operator/1
  Constant/1 -> Relational Operator/2
  Relational Operator/1 -> Error/1

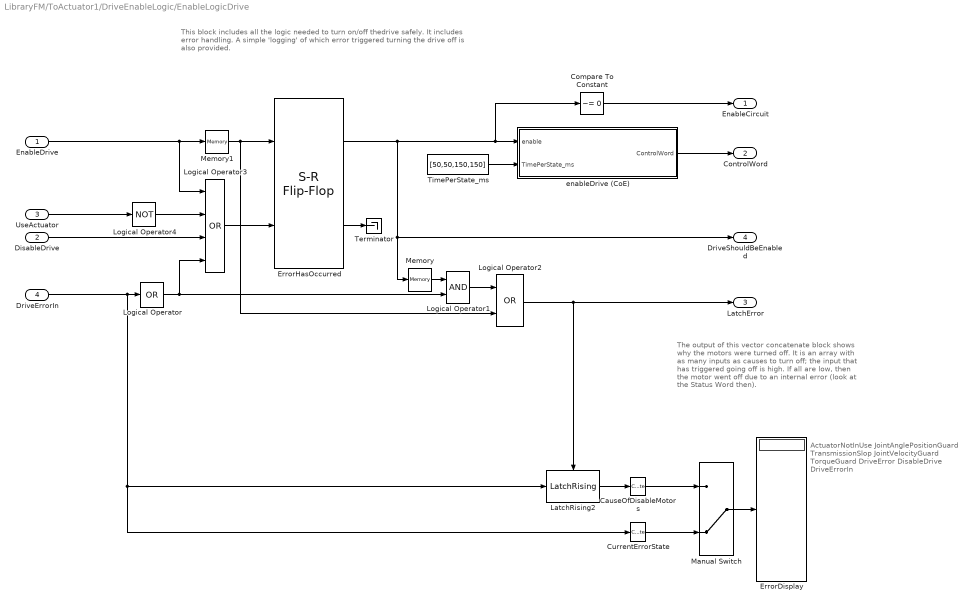
== system LibraryFM/ToActuator1/DriveEnableLogic/EnableLogicDrive ==
  note: The output of this vector concatenate block shows why the motors were turned off. It is an array with as many inputs as causes to turn off; the input that has triggered going off is high. If all are low, then the motor went off due to an internal error (look at the Status Word then).
  note: This block includes all the logic needed to turn on/off thedrive safely. It includes error handling. A simple 'logging' of which error triggered turning the drive off is also provided.
  note: ActuatorNotInUse
      | JointAnglePositionGuard
      | TransmissionSlop
      | JointVelocityGuard
      | TorqueGuard
      | DriveError
      | DisableDrive
      | DriveErrorIn
  EnableDrive : Inport
  DisableDrive : Inport  Port=2
  UseActuator : Inport  Port=3
  DriveErrorIn : Inport  Port=4
  CauseOfDisableMotors : Concatenate  NumInputs=1
  Compare To Constant : simulink/Logic and Bit Operations/Compare To Constant  relop=~=  const=0  OutDataTypeStr=boolean
  CurrentErrorState : Concatenate  NumInputs=1
  ErrorDisplay : Display
  ErrorHasOccurred : simulink_extras/Flip Flops/S-R Flip-Flop  initial_condition=0
  LatchRising2 : LibraryFM/ToActuator1/DriveEnableLogic/LatchRising
  Logical Operator : Logic  Operator=OR  Inputs=1  AllPortsSameDT=off  OutDataTypeStr=boolean
  Logical Operator1 : Logic  AllPortsSameDT=off  OutDataTypeStr=boolean
  Logical Operator2 : Logic  Operator=OR  AllPortsSameDT=off  OutDataTypeStr=boolean
  Logical Operator3 : Logic  Operator=OR  Inputs=4  AllPortsSameDT=off  OutDataTypeStr=boolean
  Logical Operator4 : Logic  Operator=NOT  Inputs=1  AllPortsSameDT=off  OutDataTypeStr=boolean
  Manual Switch : ManualSwitch  CurrentSetting=0
  Memory : Memory
  Memory1 : Memory
  Terminator : Terminator
  TimePerState_ms : Constant  Value=[50,50,150,150]
  enableDrive (CoE) : MATLAB Function  TreatAsAtomicUnit=on
  EnableCircuit : Outport
  ControlWord : Outport  Port=2
  LatchError : Outport  Port=3
  DriveShouldBeEnabled : Outport  Port=4
  wires:
  Compare To Constant/1 -> EnableCircuit/1
  Logical Operator4/1 -> Logical Operator3/2
  Manual Switch/1 -> ErrorDisplay/1
  ErrorHasOccurred/2 -> Terminator/1
  Logical Operator2/1 -> LatchRising2/Trigger, LatchError/1
  Memory1/1 -> Logical Operator2/2, ErrorHasOccurred/1
  Logical Operator/1 -> Logical Operator3/4, Logical Operator1/2
  ErrorHasOccurred/1 -> DriveShouldBeEnabled/1, Memory/1, Compare To Constant/1, enableDrive (CoE)/1(enable)
  CauseOfDisableMotors/1 -> Manual Switch/1
  LatchRising2/1 -> CauseOfDisableMotors/1
  Logical Operator1/1 -> Logical Operator2/1
  TimePerState_ms/1 -> enableDrive (CoE)/2(TimePerState_ms)
  Logical Operator3/1 -> ErrorHasOccurred/2
  Memory/1 -> Logical Operator1/1
  DriveErrorIn/1 -> CurrentErrorState/1, LatchRising2/1, Logical Operator/1
  CurrentErrorState/1 -> Manual Switch/2
  enableDrive (CoE)/1(ControlWord) -> ControlWord/1
  EnableDrive/1 -> Logical Operator3/1, Memory1/1
  UseActuator/1 -> Logical Operator4/1
  DisableDrive/1 -> Logical Operator3/3

== system LibraryFM/ToActuator1/DriveEnableLogic/LatchRising ==
  in : Inport
  Trigger : TriggerPort  VariantControl=Variant  PortDimensions=1
  out : Outport
  wires:
  in/1 -> out/1

== system LibraryFM/ToActuator1/DriveEnableLogic/8_JointVelocityGuard/LPF Diff ==
  JointPosition_rad : Inport
  Discrete Derivative : simulink/Discrete/Discrete Derivative  gainval=1.0  ICPrevScaledInput=0.0  InputProcessing=Inherited  OutMin=[]  OutMax=[]  OutDataType=fixdt(1, 16)  OutScaling=2^-10  DoSatur=off
  Freq [Hz] : Constant  Value=100  OutDataTypeStr=double
  MATLAB Function : MATLAB Function  TreatAsAtomicUnit=on
  Unit Delay : UnitDelay  SampleTime=-1
  JointVelocity_LPF_rads : Outport
  wires:
  Discrete Derivative/1 -> MATLAB Function/1(u)
  MATLAB Function/1(y) -> JointVelocity_LPF_rads/1, Unit Delay/1
  JointPosition_rad/1 -> Discrete Derivative/1
  Unit Delay/1 -> MATLAB Function/3(y_prev)
  Freq [Hz]/1 -> MATLAB Function/2(freq)

== matlab function LibraryFM/Utilities/DecodeEncoder ==
  data: Encoder_counts input; EncoderCounts_rev parameter; EncoderPosition_rad output
function EncoderPosition_rad = ...
    DecodeEncoder(Encoder_counts, EncoderCounts_rev)
%#codegen

% This block decodes the motor encoder counts to the motor angle

EncoderPosition_rad = (double(Encoder_counts) / EncoderCounts_rev * 2 * pi);

== matlab function LibraryFM/Utilities/FOAW ==
  data: x input; xdot output; sampleTime parameter; noise input
function xdot = foaw(x, sampleTime, noise)
%#codegen

SIZE = 100; % number of samples in buffer
NOISE = noise;
Ts = sampleTime;

persistent posbuffer;
persistent buffercntr;

% initialize buffer
if isempty(posbuffer)
    posbuffer = zeros(SIZE,1); % 1D case for now
    buffercntr = 0;
end

% fill buffer: shift data and add new value (loose oldest sample)
posbuffer = [posbuffer(2:end); x];
buffercntr = buffercntr + 1;
if buffercntr > SIZE, buffercntr = SIZE; end;

% if buffercntr = 1, only 1 data point is available, and you can't make a
% velocity prediction based on 1 data point. Set velocity ot 0, and return
% function
xdot = 0;
if buffercntr <= 3
    return;
end

for n = 1:buffercntr-1 % n = window size
        
    % step 2
    currentpos = posbuffer(end);

    % step 3 - calculate LS approximation of slope (hence velocity)
    b = n*sum(posbuffer(end-n:end)) - 2*sum(posbuffer(end-n:end).*(n:-1:0)');
    b = b / (Ts*n*(n+1)*(n+2)/6);

    % step 4 - check whether the line an + bn*Ts passes through all points inside the 
    % window within the uncertainty band of each point 
    jj = 0:n;
    yk_hat = currentpos-(b*jj*Ts);
    yk = posbuffer(end-jj)';
    if any(abs(yk_hat-yk) > NOISE)
        break;
    end

    xdot = b;
end

== matlab function LibraryFM/Controller_PD/inverse kinematics ==
  data: x input; xdot input; xddot input; q output size=[2 1]; Lf parameter; Lu parameter; Lb parameter; qdot output; qddot output
function [q,qdot,qddot] = IK(x,xdot,xddot,Lf,Lu,Lb)
%#codegen

% inverse dynamics
q = func_eq_IK(x(1),x(2),Lf,Lu,Lb);

% jacobians
Je = func_eq_Je(q(1),q(2),Lf,Lu,Lb);

% calculate qdot
qdot = pinv(Je)*xdot;

% calculate qddot
Jedot = func_eq_Jedot(q(1),q(2),qdot(1),qdot(2),Lf,Lu,Lb);
qddot = pinv(Je)*(xddot-Jedot*qdot);

== matlab function LibraryFM/Utilities/EncodeDesiredTorque ==
  data: MotorTorque_Des_IU output int16; JointTorque_Des_Nm input; transmissionRatio parameter; motorTorqueConstant parameter; drivePeakCurrent parameter
function MotorTorque_Des_IU = EncodeDesiredTorque(JointTorque_Des_Nm, transmissionRatio, motorTorqueConstant, drivePeakCurrent)
%#codegen
% Calculate the target torque in incremental units for a desired joint
% torque.

% compute torque at motor (negate because sign change due to transmission)
torque_motor = JointTorque_Des_Nm / transmissionRatio; 

% desired current (i_des) = torque_motor / kt (torque constant)
i_des = torque_motor / motorTorqueConstant;

% calculate the target torque in incremental units [IU], see CoE manual
% Technosoftmotion
MotorTorque_Des_IU = int16( 65520*i_des / (2*drivePeakCurrent) );

== matlab function LibraryFM/Utilities/DecodeActualTorque ==
  data: JointTorque_Act_Nm output; MotorCurrent_Act_IU input int16; transmissionRatio parameter; drivePeakCurrent parameter; motorTorqueConstant parameter
function JointTorque_Act_Nm = DecodeActualTorque(MotorCurrent_Act_IU, transmissionRatio, drivePeakCurrent, motorTorqueConstant)
%#codegen
%

% convert incremental units to motor torque value. See the technosoft CoE
% manual for the decoding
torquemotor_act = motorTorqueConstant * (double(MotorCurrent_Act_IU)*2*drivePeakCurrent / 65520);

% motor torque to joint torque (transmission). Negate due to sign change
% due to transmission.
JointTorque_Act_Nm = torquemotor_act * transmissionRatio;

== matlab function LibraryFM/Utilities/FilterFourthOrder/Filter1 ==
  data: x input; OmegaFilter input; y output; sampleTime parameter
function y = Filter2ndOrder(x, OmegaFilter, sampleTime)
%#codegen

persistent yd_prev y_prev;
if isempty(yd_prev)
    yd_prev = 0; 
    y_prev = 0; %Derivative of the above signal
end;

% Do 2nd order filtering with given omega and zeta=0.7; input of filter
% is vel_inc_sampleTime_unfilt; output is y (we assign to vel_inc_s
% later). 
if OmegaFilter==0 || isinf(OmegaFilter)
    y=x;
    y_prev=y;
    yd_prev =0;
else
    zeta = 0.7;
    ydd = OmegaFilter^2 * (x - y_prev) - 2*zeta*OmegaFilter* yd_prev;
    yd = yd_prev + ydd * sampleTime;
    y = y_prev + yd * sampleTime;

    y_prev = y; yd_prev = yd;
end;

== matlab function LibraryFM/DataToEtherCAT/FTSensorError/MATLAB Function ==
  data: ForcesTorques input; e output; MaxForcesTorques input
function e = fcn(ForcesTorques, MaxForcesTorques)

% throw error when any of the forces/torques go over a max allowable value
if any(abs(ForcesTorques) > MaxForcesTorques) 
    e = 1;
else
    e = 0;
end

== matlab function LibraryFM/StateMachineLocal/Encode system state change ==
  data: stateChanged input; state input; systemStateChanged output
function systemStateChanged  = fcn(stateChanged,state)

systemStateChanged = 0;


if stateChanged
    switch(state)
        case 201 % do calibration
            systemStateChanged = 1;
    end
end

== stateflow chart LibraryFM/StateMachineLocal/State machine ==
  state Idle
    en:
    currentState = 0;
  state Init
    en:
    currentState = 1;
    du:
    isInitialized = true;
  state Calibration
    en:
    currentState = 2;
    state JointVelLarge
    state JointVelSmall
    state DoCalibration
      en: currentState = 201;
    state CalibrationDone
      en: currentState = 299;
    (default) -> JointVelLarge
    JointVelSmall -> JointVelLarge [order 1] : [!velBelowThreshold]
    JointVelLarge -> JointVelSmall : [velBelowThreshold]
    JointVelSmall -> DoCalibration [order 2] : after(1,sec)
    DoCalibration -> CalibrationDone : after(0.1,sec)
  state Operational
    state Homing
      en:
      currentState = requestedState;
      state NotAtHome
      state AtHome
      state HomingDone
        en: currentState = 399;
      (default) -> NotAtHome
      AtHome -> NotAtHome [order 1] : [!isAtHome]
      NotAtHome -> AtHome : [isAtHome]
      AtHome -> HomingDone [order 2] : after(1,sec)
    state Run
      en: currentState = 4;
    Run -> Homing : [requestedState == 301 || requestedState == 302]
    HomingDone -> Run : [requestedState==4]
  state Error
    en: currentState=-1;
  (default) -> Idle
  Idle -> Init : [requestedState==1 || requestedState == 2]
  Init -> Calibration [order 2] : [requestedState==2]
  Init -> Idle [order 1] : [requestedState==0]
  Calibration -> Init [order 1] : [requestedState==1]
  Error -> Idle : [!fault && requestedState==0]
  Operational -> Idle [order 2] : [requestedState==0]
  Calibration -> Idle [order 2] : [requestedState==0]
  CalibrationDone -> Error [order 2] : [fault]
  CalibrationDone -> Homing [order 1] : [requestedState == 301 || requestedState == 302]
  Operational -> Error [order 1] : [fault]
  data: requestedState input double; currentState output double; fault input boolean; isInitialized local double; velBelowThreshold input boolean; isAtHome input boolean

== matlab function LibraryFM/DataFromEtherCAT/Calculate Arrange Joint and Op Space/forward kinematics/forward kinematics ==
  data: q input; x output size=[2 1]; Lf parameter; Lu parameter; Lb parameter
function x = FK(q, Lf, Lu, Lb)
%#codegen

% Calculate the endpoint position (forward kinematics)
% Note that the function func_eq_FK needs to be in the libraries/kinematis_functions folder


x = func_eq_FK(q(1),q(2),Lf,Lu,Lb);

== matlab function LibraryFM/Utilities/EndstopAndSafety/MATLAB Function ==
  data: deltaX input; v_limit output; MaxAcc input; ReturnVelocity input; ReturnVelocitySlope input
function v_limit = fcn(deltaX, MaxAcc, ReturnVelocity,ReturnVelocitySlope)
% Note: all input parameters should be positive!
% deltaX should be positive while in the 'allowed' region. If needed,
% negate the input to get it such.
%
% For the output: the v_limit is positive when in the 'allowed' region. if
% needed, negate the output to get it such.

%#codegen

if deltaX>=0
    v_limit = sqrt(2*MaxAcc * deltaX);
else
    v_limit = max ([deltaX*ReturnVelocitySlope, -ReturnVelocity]); 
end;

== matlab function LibraryFM/Utilities/EndstopAndSafety/MATLAB Function1 ==
  data: deltaX input; v_limit output; MaxAcc input; ReturnVelocity input; ReturnVelocitySlope input
function v_limit = fcn(deltaX, MaxAcc, ReturnVelocity,ReturnVelocitySlope)
% Note: all input parameters should be positive!
% deltaX should be positive while in the 'allowed' region. If needed,
% negate the input to get it such.
%
% For the output: the v_limit is positive when in the 'allowed' region. if
% needed, negate the output to get it such.

%#codegen

if deltaX>=0
    v_limit = sqrt(2*MaxAcc * deltaX);
else
    v_limit = max ([deltaX*ReturnVelocitySlope, -ReturnVelocity]); 
end;

== matlab function LibraryFM/Controller_AFFC/inverse kinematics1 ==
  data: x input; q output size=[2 1]; Lf parameter; Lu parameter; Lb parameter
function q  = IK(x,Lf,Lu,Lb)
%#codegen

% inverse dynamics
q = func_eq_IK(x(1),x(2),Lf,Lu,Lb);

== matlab function LibraryFM/Utilities/FilterFourthOrder/Filter2 ==
  data: x input; OmegaFilter input; y output; sampleTime parameter
function y = Filter2ndOrder(x, OmegaFilter, sampleTime)
%#codegen

persistent yd_prev y_prev;
if isempty(yd_prev)
    yd_prev = 0; 
    y_prev = 0; %Derivative of the above signal
end;

% Do 2nd order filtering with given omega and zeta=0.7; input of filter
% is vel_inc_sampleTime_unfilt; output is y (we assign to vel_inc_s
% later). 
if OmegaFilter==0 || isinf(OmegaFilter)
    y=x;
    y_prev=y;
    yd_prev =0;
else
    zeta = 0.7;
    ydd = OmegaFilter^2 * (x - y_prev) - 2*zeta*OmegaFilter* yd_prev;
    yd = yd_prev + ydd * sampleTime;
    y = y_prev + yd * sampleTime;

    y_prev = y; yd_prev = yd;
end;

== matlab function LibraryFM/Controller_PD/inverse kinematics1 ==
  data: x input; q output size=[2 1]; Lf parameter; Lu parameter; Lb parameter
function q  = IK(x,Lf,Lu,Lb)
%#codegen

% inverse dynamics
q = func_eq_IK(x(1),x(2),Lf,Lu,Lb);

== matlab function LibraryFM/ToActuator1/DriveEnableLogic/32_DriveError/CountHowLongEnableWasTrue ==
  data: u input; y output
function y = fcn(u)
%#codegen
%
% This block counts how many samples the input has been on (true). As soon
% as the input goes false, the counter is reset.
persistent onCounter;

if isempty(onCounter)
    onCounter = 0;
end;

if u == 1
    onCounter = onCounter + 1;
else
    % u == 0
    onCounter = 0;
end;
y = onCounter;

== matlab function LibraryFM/DriveEnableLogic1/32_DriveError/CountHowLongEnableWasTrue ==
  data: u input; y output
function y = fcn(u)
%#codegen
%
% This block counts how many samples the input has been on (true). As soon
% as the input goes false, the counter is reset.
persistent onCounter;

if isempty(onCounter)
    onCounter = 0;
end;

if u == 1
    onCounter = onCounter + 1;
else
    % u == 0
    onCounter = 0;
end;
y = onCounter;

== matlab function LibraryFM/PD + AFFC/AFFC/AFFC ==
  data: p output; t input; q input; qdot input; qddot input; e input; tau output; Lf parameter; Lu parameter; Lb parameter; w input
function [p,tau] = affc(t, q, qdot, qddot, e, Lf, Lu, Lb,w)

persistent p_;

if isempty(p_)
%     p_ = [0.00173;0.00159;0.048;0.07889;-0.00389;0.08784;-0.00474];
    p_ = zeros(7,1);
end


% jacobians
J = func_eq_Je(q(1),q(2),Lf,Lu,Lb);
Jdot = func_eq_Jedot(q(1),q(2),qdot(1),qdot(2),Lf,Lu,Lb);

% create Psi
Psi = [diag([qddot(1) qddot(2)]) J'*J*qddot+J'*Jdot*qdot [sign(qdot(1)) qdot(1); 0 0] [0 0;sign(qdot(2)) qdot(2)] ];

% learning matrix Gamma
eta = 0.95*exp(-t/150) + 0.05;

wI = w(1);
wme = w(2);
wfd = w(3);
wfs = w(4);

Gamma = eta*diag([wI wI wme wfs wfd wfs wfd]);

% update p (parameter vector)
% learning rule
dp = Gamma*Psi'*e;
p_ = p_ + dp;

% Psi = [diag([qddot(1) qddot(2)]) J'*J*qddot+J'*Jdot*qdot [ssign(qdot(1)) qdot(1); 0 0] [0 0;ssign(qdot(2)) qdot(2)] ];

% feedforward torque
tau = Psi*p_;

p = p_;

function y = ssign(u,beta)
% soft sign
if nargin == 1
    beta = 150;
end

y = 2./(1+exp(-beta*u))-1;

== matlab function LibraryFM/DataFromEtherCAT/Calculate Arrange Joint and Op Space/forward kinematics/Je ==
  data: q input; Je output size=[2 2]; Lf parameter; Lu parameter; Lb parameter
function Je = Je( q, Lf, Lu, Lb)
%#codegen

% Calculate the Jacobian for this particular device configuration.
% Note that the function func_eq_Je needs to be in the libraries/kinematis_functions folder

% jacobians
Je = func_eq_Je(q(1),q(2),Lf,Lu,Lb);

== matlab function LibraryFM/DataFromEtherCAT/Calculate Arrange Joint and Op Space/forward kinematics/Jedot ==
  data: q input; qdot input; Jedot output size=[2 2]; Lf parameter; Lu parameter; Lb parameter
function Jedot = Jedot( q, qdot, Lf, Lu, Lb)
%#codegen

% Calculate the time derivative of the Jacobian for this particular device configuration.
% Note that the function func_eq_Je needs to be in the libraries/kinematis_functions folder


% jacobians
Jedot = func_eq_Jedot(q(1),q(2),qdot(1),qdot(2),Lf,Lu,Lb);

== matlab function LibraryFM/DataFromEtherCAT/FTSensor_K6D27/CorrectOffset ==
  data: u_in input; u_out output; reset input; corrected output
function [u_out,corrected] = CorrectOffset(u_in,reset)
%#codegen

persistent data_ offset_ counter_ corrected_;
N = 1000;

% initialize
if isempty(data_)
    data_ = zeros(size(u_in,1), N);
    offset_ = zeros(size(u_in));
    counter_ = 1;
    corrected_ = 0;
end

if (counter_ <= N)
    data_(:,counter_) = u_in;
end

counter_ = counter_ + 1;
if reset
    counter_ = 1;
end

% calculate mean
if counter_ == N
    corrected_ = 1;
    offset_ = mean(data_,2);
end

corrected = corrected_;
u_out = u_in - offset_;

== matlab function LibraryFM/Controller_PD/PD + nonlin/B(q) ==
  data: y input; q input; tau output; RobotStruct parameter; Lf parameter; Lu parameter; Lb parameter
function tau = Bq(y, q, RobotStruct, Lf, Lu, Lb)
% mass matrix
phat = RobotStruct.DynModParams;

% select parameters
I1 = phat(1);
I2 = phat(2);
me = phat(3);

% jacobian
J = func_eq_Je(q(1),q(2),Lf,Lu,Lb);

% calculate joint space mass matrix;
I = diag([I1 I2]) + me*(J'*J);

% torque
tau = I*y;

== matlab function LibraryFM/DataFromEtherCAT/Calculate Arrange Joint and Op Space/IK all joints ==
  data: x input; q_all output; Lf parameter; Lu parameter; Lb parameter
function q_all = IK_all(x,Lf,Lu,Lb)
%#codegen

q_all = func_eqs_IK_all(x(1),x(2),Lf,Lu,Lb);

if any(isnan(q_all)) || any(isinf(q_all))
    q_all = zeros(5,1);
end

== matlab function LibraryFM/DataFromEtherCAT/Calculate Arrange Joint and Op Space/forward kinematics/calculate xddot ==
  data: qddot input; qdot input size=[2 1]; J input; xddot output size=[2 1]; Jdot input
function xddot = calc_xddot(qddot, qdot, J, Jdot)
%#codegen

xddot = J*qddot + Jdot*qdot;

== matlab function LibraryFM/Controller_AFFC/inverse kinematics ==
  data: x input; xdot input; xddot input; q output size=[2 1]; Lf parameter; Lu parameter; Lb parameter; qdot output; qddot output
function [q,qdot,qddot] = IK(x,xdot,xddot,Lf,Lu,Lb)
%#codegen

% inverse dynamics
q = func_eq_IK(x(1),x(2),Lf,Lu,Lb);

% jacobians
Je = func_eq_Je(q(1),q(2),Lf,Lu,Lb);

% calculate qdot
qdot = pinv(Je)*xdot;

% calculate qddot
Jedot = func_eq_Jedot(q(1),q(2),qdot(1),qdot(2),Lf,Lu,Lb);
qddot = pinv(Je)*(xddot-Jedot*qdot);

== matlab function LibraryFM/Controller_PD/PD + nonlin/nonlinear compensation ==
  data: q input; qdot input; tau output; RobotStruct parameter; Lf parameter; Lu parameter; Lb parameter
function tau = n(q, qdot, RobotStruct, Lf, Lu, Lb)
% mass matrix
phat = RobotStruct.DynModParams;

% select parameters
me = phat(3);
Fs1 = phat(4);
Fv1 = phat(5);
Fs2 = phat(6);
Fv2 = phat(7);

% jacobians
J = func_eq_Je(q(1),q(2),Lf,Lu,Lb);
Jdot = func_eq_Jedot(q(1),q(2),qdot(1),qdot(2),Lf,Lu,Lb);

% calculate joint space mass matrix;
p = [me;Fs1;Fv1;Fs2;Fv2];

% psi 
Psi = [(J'*Jdot)*qdot [ssign(qdot(1)) qdot(1); 0 0] [0 0; ssign(qdot(2)) qdot(2)]];

% torque
tau = Psi*p;

function x = ssign(u,b)
%% x = ssign(u,b)
% soft sign
if nargin < 2
    b = 150;
end

x = 2./(1+exp(-b*u))-1;

== matlab function LibraryFM/LPF Diff/MATLAB Function ==
  data: u input; freq input; y output; y_prev input; sampleTime parameter
function y = fcn(u,freq,y_prev,sampleTime)
tau = 1/(freq*2*pi);
a = sampleTime/(sampleTime + tau);
y = y_prev*(1-a) + a*u;
